simulink model "Arti_DeltaSM_Control_Fricc"  (R2014a)
settings: Solver=ode15s  StartTime=0.0  StopTime=6  FixedStep=0.0005  RelTol=1e-3
PreLoadFcn:
  | Fs=0.001;
  | Fc=0.0005;
undefined symbols (not defined in the file or in its folder): X, Y, Z
libraries: sm_lib x238, Fricciones x15, nesl_utility x10, simulink x3
(part 1 of 6)
Description:
  | Modelo de un robot tipo Delta, con:
  | -Fricción en las articulaciones
  | -Con interpolador de orden 5 en el espacio operacional.
  | -Cinematica inversa
  | -Sigue una trayectoria dada de pick and place con un control, y se obtiene la posicion final del efector.
  | -Tiene un control PID
  | 
  | le falta caracterizacion de los motores
settings Model: Creator=Sebastian Serna Palleja  LastModifiedBy=Sebastian
settings Model: ModifiedComment=|
  | Sebastian -- Mon Apr 11 18:51:16 2016 -- Version 1.58
  | actualizacion de pesos
settings Model: ModifiedHistory=|
  | Sebastian -- Mon Apr 11 18:51:16 2016 -- Version 1.58
  | actualizacion de pesos
  | 
  | Sebastian -- Sat Apr 09 23:12:04 2016 -- Version 1.56
  | Modelo organizado
settings SolverCC: MaxConsecutiveMinStep=4

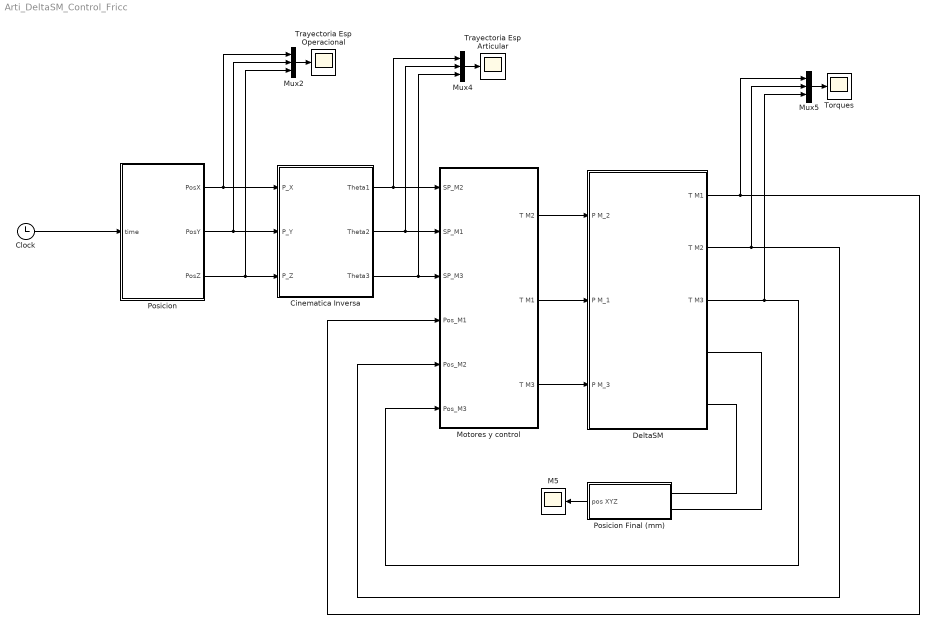
== system Arti_DeltaSM_Control_Fricc ==
  Cinematica Inversa : Subsystem
  Clock : Clock
  DeltaSM : Subsystem
  M5 : Scope
      settings: TimeRange=2  YMin=-450  YMax=50  SaveName=salida1
  Motores y control : Subsystem
  Mux2 : Mux  Inputs=3
  Mux4 : Mux  Inputs=3
  Mux5 : Mux  Inputs=3
  "Posicion " : MATLAB Function  TreatAsAtomicUnit=on
  Posicion Final (mm) : Subsystem
  Torques : Scope
      settings: SaveName=ScopeData11
  Trayectoria Esp Articular : Scope
      settings: SaveName=ScopeData9
  Trayectoria Esp Operacional : Scope
      settings: SaveName=ScopeData4
  wires:
  Posicion Final (mm)/1(pos XYZ) -> M5/1
  Clock/1 -> "Posicion "/1(time)
  Motores y control/3(T M3) -> DeltaSM/3(P M_3)
  Motores y control/2(T M1) -> DeltaSM/2(P M_1)
  Motores y control/1(T M2) -> DeltaSM/1(P M_2)
  Mux2/1 -> Trayectoria Esp Operacional/1
  "Posicion "/3(PosZ) -> Mux2/3, Cinematica Inversa/3(P_Z)
  "Posicion "/2(PosY) -> Mux2/2, Cinematica Inversa/2(P_Y)
  "Posicion "/1(PosX) -> Mux2/1, Cinematica Inversa/1(P_X)
  Mux4/1 -> Trayectoria Esp Articular/1
  Cinematica Inversa/3(Theta3) -> Mux4/3, Motores y control/3(SP_M3)
  Cinematica Inversa/2(Theta2) -> Mux4/2, Motores y control/2(SP_M1)
  Cinematica Inversa/1(Theta1) -> Mux4/1, Motores y control/1(SP_M2)
  Mux5/1 -> Torques/1
  DeltaSM/3(T M3) -> Mux5/3, Motores y control/6(Pos_M3)
  DeltaSM/2(T M2) -> Mux5/2, Motores y control/5(Pos_M2)
  DeltaSM/1(T M1) -> Mux5/1, Motores y control/4(Pos_M1)
  connections:
  Posicion Final (mm)/LConn2 -- DeltaSM/RConn1
  Posicion Final (mm)/LConn1 -- DeltaSM/RConn2

== system Arti_DeltaSM_Control_Fricc/Cinematica Inversa ==
  P_X : Inport
  P_Y : Inport  Port=2
  P_Z : Inport  Port=3
  Cinematica Inversa : MATLAB Function  TreatAsAtomicUnit=on
  G_1 : Gain
  G_2 : Gain
  G_3 : Gain  Gain=-1
  Retardo1 : TransportDelay  DelayTime=0.01
  Retardo2 : TransportDelay  DelayTime=0.01
  Retardo3 : TransportDelay  DelayTime=0.01
  Theta1 : Outport
  Theta2 : Outport  Port=2
  Theta3 : Outport  Port=3
  wires:
  P_X/1 -> Cinematica Inversa/1(Px)
  P_Y/1 -> Cinematica Inversa/2(Py)
  Cinematica Inversa/3(ThetaM3) -> G_3/1, Retardo1/1
  Retardo2/1 -> Cinematica Inversa/5(AntThetaM2)
  Retardo3/1 -> Cinematica Inversa/4(AntThetaM1)
  Retardo1/1 -> Cinematica Inversa/6(AntThetaM3)
  Cinematica Inversa/1(ThetaM1) -> G_1/1, Retardo3/1
  Cinematica Inversa/2(ThetaM2) -> G_2/1, Retardo2/1
  G_1/1 -> Theta1/1
  G_2/1 -> Theta2/1
  G_3/1 -> Theta3/1
  P_Z/1 -> Cinematica Inversa/3(Pz)

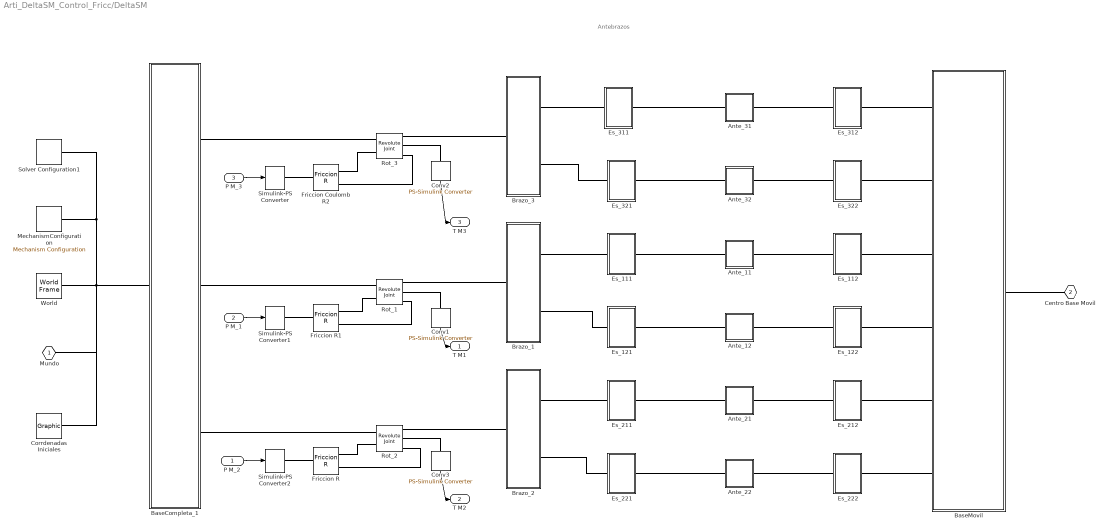
== system Arti_DeltaSM_Control_Fricc/DeltaSM ==
  note: Antebrazos
  P M_2 : Inport
  P M_1 : Inport  Port=2
  P M_3 : Inport  Port=3
  Ante_11 : Subsystem
  Ante_12 : Subsystem
  Ante_21 : Subsystem
  Ante_22 : Subsystem
  Ante_31 : Subsystem
  Ante_32 : Subsystem
  BaseCompleta_1 : Subsystem
  BaseMovil : Subsystem
  Brazo_1 : Subsystem
  Brazo_2 : Subsystem
  Brazo_3 : Subsystem
  Conv1 : nesl_utility/PS-Simulink Converter  PhysicalDomain=network_engine_domain  SubClassName=ps_output  LeftPortType=input  RightPortType=output  PseudoPeriodic=off  Frequencies=[]  Unit=rad  AffineConversion=off
  Conv2 : nesl_utility/PS-Simulink Converter  PhysicalDomain=network_engine_domain  SubClassName=ps_output  LeftPortType=input  RightPortType=output  PseudoPeriodic=off  Frequencies=[]  Unit=rad  AffineConversion=off
  Conv3 : nesl_utility/PS-Simulink Converter  PhysicalDomain=network_engine_domain  SubClassName=ps_output  LeftPortType=input  RightPortType=output  PseudoPeriodic=off  Frequencies=[]  Unit=rad  AffineConversion=off
  "Corrdenadas Iniciales " : sm_lib/Body Elements/Graphic  GraphicType=Marker  MarkerShape=Frame  MarkerSize=25  MarkerSizeUnits=m  GraphicVisPropType=SimpleVisualProperties  GraphicDiffuseColor=[0.0 0.0 0.0]  GraphicSpecularColor=[0.2 0.2 0.2]  GraphicAmbientColor=[0.5 0.5 0.5]  GraphicEmissiveColor=[0.0 0.0 0.0 1.0]  GraphicShininess=24.0  GraphicOpacity=1.0  BlockFunction=simmechanics.library.body_elements.graphic
  Es_111 : Subsystem
  Es_112 : Subsystem
  Es_121 : Subsystem
  Es_122 : Subsystem
  Es_211 : Subsystem
  Es_212 : Subsystem
  Es_221 : Subsystem
  Es_222 : Subsystem
  Es_311 : Subsystem
  Es_312 : Subsystem
  Es_321 : Subsystem
  Es_322 : Subsystem
  Friccion Coulomb R2 : Fricciones/Friccion R
  Friccion R : Fricciones/Friccion R
  Friccion R1 : Fricciones/Friccion R
  MechanismConfiguration : sm_lib/Utilities/Mechanism Configuration  UniformGravity=Constant  GravityVector=[0 0 -9.81]  GravityUnits=m/s^2  LinearizationDelta=0.001  BlockFunction=simmechanics.library.utilities.mechanism_configuration
  Rot_1 : sm_lib/Joints/Revolute Joint  SenseConstraintForce=off  SenseConstraintForceX=off  SenseConstraintForceY=off  SenseConstraintForceZ=off  SenseConstraintTorque=off  SenseConstraintTorqueX=off  SenseConstraintTorqueY=off  SenseConstraintTorqueZ=off  SenseTotalForce=off  SenseTotalForceX=off  SenseTotalForceY=off  SenseTotalForceZ=off  SenseTotalTorque=off  SenseTotalTorqueX=off  SenseTotalTorqueY=off  SenseTotalTorqueZ=off  CompositeWrenchDir=FollowerOnBase  CompositeWrenchFrame=BaseFrame  EquilibriumPosition=0  EquilibriumPositionUnits=rad  SpringStiffness=0  SpringStiffnessUnits=m*N/rad  DampingCoefficient=0  DampingCoefficientUnits=m*s*N/rad  TorqueActuationMode=InputTorque  MotionActuationMode=ComputedMotion  SensePosition=on  SenseVelocity=on  SenseAcceleration=off  SenseTorqueForce=off  PositionTargetValue=90  PositionTargetValueUnits=deg  PositionTargetSpecify=on  PositionTargetPriority=High  VelocityTargetValue=0  VelocityTargetValueUnits=deg/s  VelocityTargetSpecify=off  VelocityTargetPriority=High  BlockFunction=simmechanics.library.joints.revolute_joint
  Rot_2 : sm_lib/Joints/Revolute Joint  SenseConstraintForce=off  SenseConstraintForceX=off  SenseConstraintForceY=off  SenseConstraintForceZ=off  SenseConstraintTorque=off  SenseConstraintTorqueX=off  SenseConstraintTorqueY=off  SenseConstraintTorqueZ=off  SenseTotalForce=off  SenseTotalForceX=off  SenseTotalForceY=off  SenseTotalForceZ=off  SenseTotalTorque=off  SenseTotalTorqueX=off  SenseTotalTorqueY=off  SenseTotalTorqueZ=off  CompositeWrenchDir=FollowerOnBase  CompositeWrenchFrame=BaseFrame  EquilibriumPosition=0  EquilibriumPositionUnits=rad  SpringStiffness=0  SpringStiffnessUnits=m*N/rad  DampingCoefficient=0  DampingCoefficientUnits=m*s*N/rad  TorqueActuationMode=InputTorque  MotionActuationMode=ComputedMotion  SensePosition=on  SenseVelocity=on  SenseAcceleration=off  SenseTorqueForce=off  PositionTargetValue=90  PositionTargetValueUnits=deg  PositionTargetSpecify=on  PositionTargetPriority=High  VelocityTargetValue=0  VelocityTargetValueUnits=deg/s  VelocityTargetSpecify=off  VelocityTargetPriority=High  BlockFunction=simmechanics.library.joints.revolute_joint
  Rot_3 : sm_lib/Joints/Revolute Joint  SenseConstraintForce=off  SenseConstraintForceX=off  SenseConstraintForceY=off  SenseConstraintForceZ=off  SenseConstraintTorque=off  SenseConstraintTorqueX=off  SenseConstraintTorqueY=off  SenseConstraintTorqueZ=off  SenseTotalForce=off  SenseTotalForceX=off  SenseTotalForceY=off  SenseTotalForceZ=off  SenseTotalTorque=off  SenseTotalTorqueX=off  SenseTotalTorqueY=off  SenseTotalTorqueZ=off  CompositeWrenchDir=FollowerOnBase  CompositeWrenchFrame=BaseFrame  EquilibriumPosition=0  EquilibriumPositionUnits=rad  SpringStiffness=0  SpringStiffnessUnits=m*N/rad  DampingCoefficient=0  DampingCoefficientUnits=m*s*N/rad  TorqueActuationMode=InputTorque  MotionActuationMode=ComputedMotion  SensePosition=on  SenseVelocity=on  SenseAcceleration=off  SenseTorqueForce=off  PositionTargetValue=-90  PositionTargetValueUnits=deg  PositionTargetSpecify=on  PositionTargetPriority=High  VelocityTargetValue=0  VelocityTargetValueUnits=deg/s  VelocityTargetSpecify=off  VelocityTargetPriority=High  BlockFunction=simmechanics.library.joints.revolute_joint
  Simulink-PS Converter : nesl_utility/Simulink-PS Converter  PhysicalDomain=network_engine_domain  SubClassName=ps_input  LeftPortType=input  RightPortType=output  PseudoPeriodic=off  Frequencies=[]  NoiseDistribution=none  NoiseParameters=[]  Unit=N*m  AffineConversion=off  InputFiltering=off  SimscapeFilterOrder=1  InputFilterTimeConstant=0.001  UdotUserProvided=1
  Simulink-PS Converter1 : nesl_utility/Simulink-PS Converter  PhysicalDomain=network_engine_domain  SubClassName=ps_input  LeftPortType=input  RightPortType=output  PseudoPeriodic=off  Frequencies=[]  NoiseDistribution=none  NoiseParameters=[]  Unit=N*m  AffineConversion=off  InputFiltering=off  SimscapeFilterOrder=1  InputFilterTimeConstant=0.001  UdotUserProvided=1
  Simulink-PS Converter2 : nesl_utility/Simulink-PS Converter  PhysicalDomain=network_engine_domain  SubClassName=ps_input  LeftPortType=input  RightPortType=output  PseudoPeriodic=off  Frequencies=[]  NoiseDistribution=none  NoiseParameters=[]  Unit=N*m  AffineConversion=off  InputFiltering=off  SimscapeFilterOrder=1  InputFilterTimeConstant=0.001  UdotUserProvided=1
  Solver Configuration1 : nesl_utility/Solver Configuration  PhysicalDomain=network_engine_domain  SubClassName=solver  LeftPortType=input  RightPortType=generic  Accelerate=off  Tones=[]  Harmonics=[]  SimulateNoise=off  Profile=off  UseLocalSampling=off  EnableSwitchedLinearOptims=on  FrequencyDomain=off  UseCCode=off  RelTol=0.001  AbsTol=1e-06  MinStep=1e-09  ToWorkspace=off  DoDC=on  ResidualTolerance=1e-09  UseLocalSolver=off  LocalSolverChoice=NE_BACKWARD_EULER_ADVANCER  LocalSolverSampleTime=0.00001  DoFixedCost=off  MaxNonlinIter=30  MaxModeIter=2  LinearAlgebra=Full  DelaysMemoryBudget=2048  AutomaticFiltering=on  FilteringTimeConstant=0.001
  World : sm_lib/Frames and Transforms/World Frame  BlockFunction=simmechanics.library.frames_transforms.world_frame
  Mundo : PMIOPort  Port=1  Side=Right
  Centro Base Movil : PMIOPort  Priority=1  Port=2  Side=Right
  T M1 : Outport
  T M2 : Outport  Port=2
  T M3 : Outport  Port=3
  wires:
  Conv2/1 -> T M3/1
  Conv1/1 -> T M1/1
  Conv3/1 -> T M2/1
  P M_1/1 -> Simulink-PS Converter1/1
  P M_3/1 -> Simulink-PS Converter/1
  P M_2/1 -> Simulink-PS Converter2/1
  connections:
  BaseCompleta_1/RConn2 -- Rot_1/LConn1
  Brazo_2/LConn1 -- Rot_2/RConn1
  BaseCompleta_1/RConn1 -- Rot_3/LConn1
  Brazo_3/LConn1 -- Rot_3/RConn1
  Brazo_1/LConn1 -- Rot_1/RConn1
  BaseCompleta_1/RConn3 -- Rot_2/LConn1
  Conv2/LConn1 -- Rot_3/RConn2
  Conv1/LConn1 -- Rot_1/RConn2
  Conv3/LConn1 -- Rot_2/RConn2
  BaseMovil/RConn1 -- Centro Base Movil/RConn1
  Friccion R1/LConn1 -- Simulink-PS Converter1/RConn1
  Friccion R1/RConn1 -- Rot_1/LConn2
  Friccion R1/RConn2 -- Rot_1/RConn3
  Friccion R/RConn2 -- Rot_2/RConn3
  Rot_3/RConn3 -- Friccion Coulomb R2/RConn2
  Friccion R/LConn1 -- Simulink-PS Converter2/RConn1
  Friccion R/RConn1 -- Rot_2/LConn2
  Friccion Coulomb R2/RConn1 -- Rot_3/LConn2
  Simulink-PS Converter/RConn1 -- Friccion Coulomb R2/LConn1
  Ante_11/RConn1 -- Es_112/LConn1
  Ante_22/LConn1 -- Es_221/RConn1
  Ante_31/RConn1 -- Es_312/LConn1
  Brazo_1/RConn2 -- Es_121/LConn1
  Brazo_3/RConn2 -- Es_321/LConn1
  Ante_32/RConn1 -- Es_322/LConn1
  Ante_22/RConn1 -- Es_222/LConn1
  Brazo_3/RConn1 -- Es_311/LConn1
  Ante_21/LConn1 -- Es_211/RConn1
  Ante_12/RConn1 -- Es_122/LConn1
  Ante_31/LConn1 -- Es_311/RConn1
  Ante_11/LConn1 -- Es_111/RConn1
  Ante_21/RConn1 -- Es_212/LConn1
  BaseMovil/LConn1 -- Es_312/RConn1
  BaseMovil/LConn5 -- Es_212/RConn1
  BaseMovil/LConn6 -- Es_222/RConn1
  Ante_32/LConn1 -- Es_321/RConn1
  BaseMovil/LConn3 -- Es_112/RConn1
  Brazo_2/RConn2 -- Es_221/LConn1
  BaseMovil/LConn4 -- Es_122/RConn1
  BaseMovil/LConn2 -- Es_322/RConn1
  Brazo_2/RConn1 -- Es_211/LConn1
  Ante_12/LConn1 -- Es_121/RConn1
  Brazo_1/RConn1 -- Es_111/LConn1
  Solver Configuration1/RConn1 -- MechanismConfiguration/RConn1 -- BaseCompleta_1/LConn1 -- Mundo/RConn1 -- "Corrdenadas Iniciales "/RConn1 -- World/RConn1

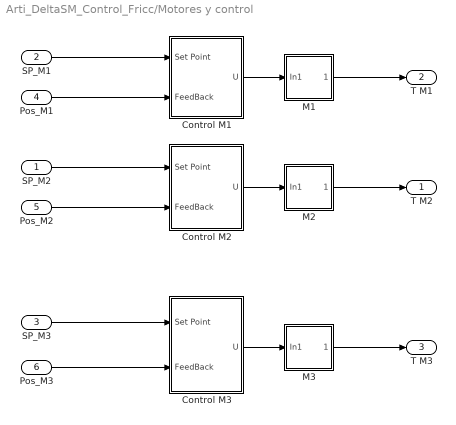
== system Arti_DeltaSM_Control_Fricc/Motores y control ==
  SP_M2 : Inport
  SP_M1 : Inport  Port=2
  SP_M3 : Inport  Port=3
  Pos_M1 : Inport  Port=4
  Pos_M2 : Inport  Port=5
  Pos_M3 : Inport  Port=6
  Control M1 : Subsystem
  Control M2 : Subsystem
  Control M3 : Subsystem
  M1 : Subsystem
  M2 : Subsystem
  M3 : Subsystem
  T M2 : Outport
  T M1 : Outport  Port=2
  T M3 : Outport  Port=3
  wires:
  SP_M2/1 -> Control M2/1(Set Point)
  Pos_M2/1 -> Control M2/2(FeedBack)
  SP_M1/1 -> Control M1/1(Set Point)
  Pos_M1/1 -> Control M1/2(FeedBack)
  Control M2/1(U) -> M2/1(In1)
  Control M1/1(U) -> M1/1(In1)
  Control M3/1(U) -> M3/1(In1)
  SP_M3/1 -> Control M3/1(Set Point)
  Pos_M3/1 -> Control M3/2(FeedBack)
  M1/1(Out1) -> T M1/1
  M2/1(Out1) -> T M2/1
  M3/1(Out1) -> T M3/1

== system Arti_DeltaSM_Control_Fricc/Posicion Final (mm) ==
  M1 : Scope
      settings: SaveName=ScopeData7
  M2 : Scope
      settings: SaveName=ScopeData8
  "M3 " : Scope
      settings: SaveName=ScopeData6
  Mux : Mux  Inputs=3
  Pos X Converter : nesl_utility/PS-Simulink Converter  PhysicalDomain=network_engine_domain  SubClassName=ps_output  LeftPortType=input  RightPortType=output  PseudoPeriodic=off  Frequencies=[]  Unit=mm  AffineConversion=off
  Pos Y Converter1 : nesl_utility/PS-Simulink Converter  PhysicalDomain=network_engine_domain  SubClassName=ps_output  LeftPortType=input  RightPortType=output  PseudoPeriodic=off  Frequencies=[]  Unit=mm  AffineConversion=off
  Pos Z Converter2 : nesl_utility/PS-Simulink Converter  PhysicalDomain=network_engine_domain  SubClassName=ps_output  LeftPortType=input  RightPortType=output  PseudoPeriodic=off  Frequencies=[]  Unit=mm  AffineConversion=off
  Transform Sensor : sm_lib/Frames and Transforms/Transform Sensor  MeasurementFrame=World  SenseAngle=off  SenseAxis=off  SenseAngle1=off  SenseAngle2=off  SenseAngle3=off  SenseQ=off  SenseR=off  SenseOmegaX=off  SenseOmegaY=off  SenseOmegaZ=off  SenseOmega1=off  SenseOmega2=off  SenseOmega3=off  SenseQDot=off  SenseRDot=off  SenseAlphaX=off  SenseAlphaY=off  SenseAlphaZ=off  SenseAlpha1=off  SenseAlpha2=off  SenseAlpha3=off  SenseQDDot=off  SenseRDDot=off  SenseX=on  SenseY=on  SenseZ=on  SenseRad=off  SenseAzim=off  SenseDist=off  SenseInc=off  SenseXDot=off  SenseYDot=off  SenseZDot=off  SenseRadDot=off  SenseAzimDot=off  SenseDistDot=off  SenseIncDot=off  SenseXDDot=off  SenseYDDot=off  SenseZDDot=off  SenseRadDDot=off  SenseAzimDDot=off  SenseDistDDot=off  SenseIncDDot=off  BlockFunction=simmechanics.library.frames_transforms.transform_sensor
  Centro Base Movil : PMIOPort  Port=1  Side=Left
  world : PMIOPort  Port=2  Side=Left
  pos XYZ : Outport
  wires:
  Pos Z Converter2/1 -> M2/1, Mux/3
  Mux/1 -> pos XYZ/1
  Pos Y Converter1/1 -> Mux/2, M1/1
  Pos X Converter/1 -> "M3 "/1, Mux/1
  connections:
  world/RConn1 -- Transform Sensor/LConn1
  Pos Z Converter2/LConn1 -- Transform Sensor/RConn4
  Transform Sensor/RConn2 -- Pos X Converter/LConn1
  Pos Y Converter1/LConn1 -- Transform Sensor/RConn3
  Centro Base Movil/RConn1 -- Transform Sensor/RConn1

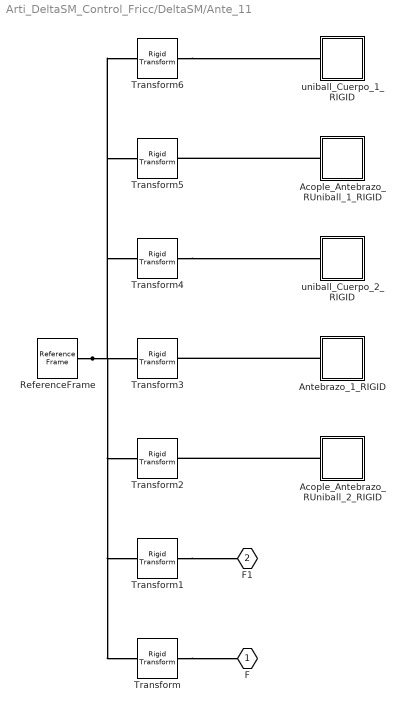
== system Arti_DeltaSM_Control_Fricc/DeltaSM/Ante_11 ==
  Acople_Antebrazo_RUniball_1_RIGID : Subsystem
  Acople_Antebrazo_RUniball_2_RIGID : Subsystem
  Antebrazo_1_RIGID : Subsystem
  ReferenceFrame : sm_lib/Frames and Transforms/Reference Frame  BlockFunction=simmechanics.library.frames_transforms.reference_frame
  Transform : sm_lib/Frames and Transforms/Rigid Transform  TranslationMethod=Cartesian  TranslationLengthUnit=mm  TranslationStandardAxis=+Z  TranslationStandardOffset=0  TranslationCartesianOffset=[-16.089268306127384 11.758961591624281 40.649351392904187]  TranslationROffset=0  TranslationROffsetUnits=m  TranslationZOffset=0  TranslationZOffsetUnits=m  TranslationThetaOffset=0  TranslationThetaOffsetUnits=deg  RotationMethod=ArbitraryAxis  RotationAngleUnits=rad  RotationStandardAxis=+Z  RotationAngle=0  RotationArbitraryAxis=[0 0 0]  FollAlignAxisA=+X  BaseAlignAxisA=+Y  FollAlignAxisB=+Y  BaseAlignAxisB=+Z  BlockFunction=simmechanics.library.frames_transforms.rigid_transform
  Transform1 : sm_lib/Frames and Transforms/Rigid Transform  TranslationMethod=Cartesian  TranslationLengthUnit=mm  TranslationStandardAxis=+Z  TranslationStandardOffset=0  TranslationCartesianOffset=[-16.089268306127369 -263.24103840837563 40.649351392904151]  TranslationROffset=0  TranslationROffsetUnits=m  TranslationZOffset=0  TranslationZOffsetUnits=m  TranslationThetaOffset=0  TranslationThetaOffsetUnits=deg  RotationMethod=ArbitraryAxis  RotationAngleUnits=rad  RotationStandardAxis=+Z  RotationAngle=0  RotationArbitraryAxis=[0 0 0]  FollAlignAxisA=+X  BaseAlignAxisA=+Y  FollAlignAxisB=+Y  BaseAlignAxisB=+Z  BlockFunction=simmechanics.library.frames_transforms.rigid_transform
  Transform2 : sm_lib/Frames and Transforms/Rigid Transform  TranslationMethod=Cartesian  TranslationLengthUnit=mm  TranslationStandardAxis=+Z  TranslationStandardOffset=0  TranslationCartesianOffset=[-16.089268306127376 -51.741038408375687 40.649351392904165]  TranslationROffset=0  TranslationROffsetUnits=m  TranslationZOffset=0  TranslationZOffsetUnits=m  TranslationThetaOffset=0  TranslationThetaOffsetUnits=deg  RotationMethod=ArbitraryAxis  RotationAngleUnits=rad  RotationStandardAxis=+Z  RotationAngle=2.7352803968007873  RotationArbitraryAxis=[-0.2059979679735047 0.69194105138761164 0.69194105138761175]  FollAlignAxisA=+X  BaseAlignAxisA=+Y  FollAlignAxisB=+Y  BaseAlignAxisB=+Z  BlockFunction=simmechanics.library.frames_transforms.rigid_transform
  Transform3 : sm_lib/Frames and Transforms/Rigid Transform  TranslationMethod=Cartesian  TranslationLengthUnit=mm  TranslationStandardAxis=+Z  TranslationStandardOffset=0  TranslationCartesianOffset=[-16.089268306127384 -227.74103840837574 40.64935139290418]  TranslationROffset=0  TranslationROffsetUnits=m  TranslationZOffset=0  TranslationZOffsetUnits=m  TranslationThetaOffset=0  TranslationThetaOffsetUnits=deg  RotationMethod=ArbitraryAxis  RotationAngleUnits=rad  RotationStandardAxis=+Z  RotationAngle=2.7352803968007873  RotationArbitraryAxis=[-0.2059979679735047 0.69194105138761164 0.69194105138761175]  FollAlignAxisA=+X  BaseAlignAxisA=+Y  FollAlignAxisB=+Y  BaseAlignAxisB=+Z  BlockFunction=simmechanics.library.frames_transforms.rigid_transform
  Transform4 : sm_lib/Frames and Transforms/Rigid Transform  TranslationMethod=Cartesian  TranslationLengthUnit=mm  TranslationStandardAxis=+Z  TranslationStandardOffset=0  TranslationCartesianOffset=[-16.089268306127369 -263.24103840837563 40.649351392904151]  TranslationROffset=0  TranslationROffsetUnits=m  TranslationZOffset=0  TranslationZOffsetUnits=m  TranslationThetaOffset=0  TranslationThetaOffsetUnits=deg  RotationMethod=ArbitraryAxis  RotationAngleUnits=rad  RotationStandardAxis=+Z  RotationAngle=3.1415926535897931  RotationArbitraryAxis=[-1.1188966420050406e-16 0 1]  FollAlignAxisA=+X  BaseAlignAxisA=+Y  FollAlignAxisB=+Y  BaseAlignAxisB=+Z  BlockFunction=simmechanics.library.frames_transforms.rigid_transform
  Transform5 : sm_lib/Frames and Transforms/Rigid Transform  TranslationMethod=Cartesian  TranslationLengthUnit=mm  TranslationStandardAxis=+Z  TranslationStandardOffset=0  TranslationCartesianOffset=[-16.089268306127391 -199.7410384083758 40.64935139290418]  TranslationROffset=0  TranslationROffsetUnits=m  TranslationZOffset=0  TranslationZOffsetUnits=m  TranslationThetaOffset=0  TranslationThetaOffsetUnits=deg  RotationMethod=ArbitraryAxis  RotationAngleUnits=rad  RotationStandardAxis=+Z  RotationAngle=2.7352803968007873  RotationArbitraryAxis=[0.2059979679735047 0.69194105138761164 -0.69194105138761175]  FollAlignAxisA=+X  BaseAlignAxisA=+Y  FollAlignAxisB=+Y  BaseAlignAxisB=+Z  BlockFunction=simmechanics.library.frames_transforms.rigid_transform
  Transform6 : sm_lib/Frames and Transforms/Rigid Transform  TranslationMethod=Cartesian  TranslationLengthUnit=mm  TranslationStandardAxis=+Z  TranslationStandardOffset=0  TranslationCartesianOffset=[-16.089268306127376 11.758961591624317 40.649351392904165]  TranslationROffset=0  TranslationROffsetUnits=m  TranslationZOffset=0  TranslationZOffsetUnits=m  TranslationThetaOffset=0  TranslationThetaOffsetUnits=deg  RotationMethod=None  RotationAngleUnits=deg  RotationStandardAxis=+Z  RotationAngle=0  RotationArbitraryAxis=[0 0 1]  FollAlignAxisA=+X  BaseAlignAxisA=+Y  FollAlignAxisB=+Y  BaseAlignAxisB=+Z  BlockFunction=simmechanics.library.frames_transforms.rigid_transform
  uniball_Cuerpo_1_RIGID : Subsystem
  uniball_Cuerpo_2_RIGID : Subsystem
  F : PMIOPort  Port=1  Side=Left
  F1 : PMIOPort  Port=2  Side=Right
  connections:
  ReferenceFrame/RConn1 -- Transform/LConn1 -- Transform1/LConn1 -- Transform2/LConn1 -- Transform3/LConn1 -- Transform4/LConn1 -- Transform5/LConn1 -- Transform6/LConn1
  Transform/RConn1 -- F/RConn1
  Transform1/RConn1 -- F1/RConn1
  Acople_Antebrazo_RUniball_2_RIGID/LConn1 -- Transform2/RConn1
  Antebrazo_1_RIGID/LConn1 -- Transform3/RConn1
  Transform4/RConn1 -- uniball_Cuerpo_2_RIGID/LConn1
  Acople_Antebrazo_RUniball_1_RIGID/LConn1 -- Transform5/RConn1
  Transform6/RConn1 -- uniball_Cuerpo_1_RIGID/LConn1

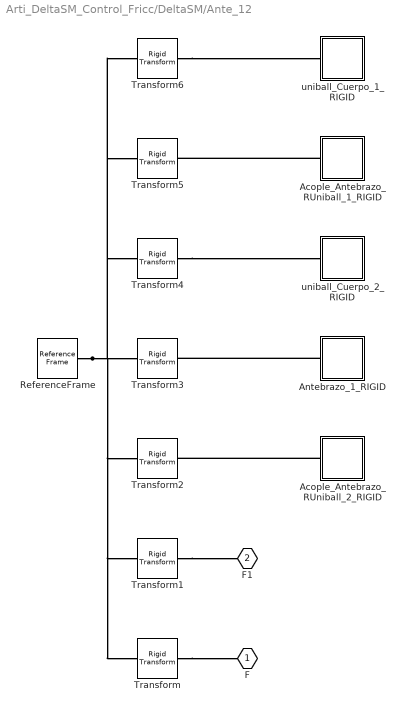
== system Arti_DeltaSM_Control_Fricc/DeltaSM/Ante_12 ==
  Acople_Antebrazo_RUniball_1_RIGID : Subsystem
  Acople_Antebrazo_RUniball_2_RIGID : Subsystem
  Antebrazo_1_RIGID : Subsystem
  ReferenceFrame : sm_lib/Frames and Transforms/Reference Frame  BlockFunction=simmechanics.library.frames_transforms.reference_frame
  Transform : sm_lib/Frames and Transforms/Rigid Transform  TranslationMethod=Cartesian  TranslationLengthUnit=mm  TranslationStandardAxis=+Z  TranslationStandardOffset=0  TranslationCartesianOffset=[-16.089268306127394 11.758961591624296 40.64935139290418]  TranslationROffset=0  TranslationROffsetUnits=m  TranslationZOffset=0  TranslationZOffsetUnits=m  TranslationThetaOffset=0  TranslationThetaOffsetUnits=deg  RotationMethod=ArbitraryAxis  RotationAngleUnits=rad  RotationStandardAxis=+Z  RotationAngle=0  RotationArbitraryAxis=[0 0 0]  FollAlignAxisA=+X  BaseAlignAxisA=+Y  FollAlignAxisB=+Y  BaseAlignAxisB=+Z  BlockFunction=simmechanics.library.frames_transforms.rigid_transform
  Transform1 : sm_lib/Frames and Transforms/Rigid Transform  TranslationMethod=Cartesian  TranslationLengthUnit=mm  TranslationStandardAxis=+Z  TranslationStandardOffset=0  TranslationCartesianOffset=[-16.089268306127391 -263.24103840837574 40.649351392904165]  TranslationROffset=0  TranslationROffsetUnits=m  TranslationZOffset=0  TranslationZOffsetUnits=m  TranslationThetaOffset=0  TranslationThetaOffsetUnits=deg  RotationMethod=ArbitraryAxis  RotationAngleUnits=rad  RotationStandardAxis=+Z  RotationAngle=0  RotationArbitraryAxis=[0 0 0]  FollAlignAxisA=+X  BaseAlignAxisA=+Y  FollAlignAxisB=+Y  BaseAlignAxisB=+Z  BlockFunction=simmechanics.library.frames_transforms.rigid_transform
  Transform2 : sm_lib/Frames and Transforms/Rigid Transform  TranslationMethod=Cartesian  TranslationLengthUnit=mm  TranslationStandardAxis=+Z  TranslationStandardOffset=0  TranslationCartesianOffset=[-16.089268306127362 -51.741038408375672 40.64935139290418]  TranslationROffset=0  TranslationROffsetUnits=m  TranslationZOffset=0  TranslationZOffsetUnits=m  TranslationThetaOffset=0  TranslationThetaOffsetUnits=deg  RotationMethod=ArbitraryAxis  RotationAngleUnits=rad  RotationStandardAxis=+Z  RotationAngle=2.7352803968007873  RotationArbitraryAxis=[-0.20599796797350473 0.69194105138761164 0.69194105138761175]  FollAlignAxisA=+X  BaseAlignAxisA=+Y  FollAlignAxisB=+Y  BaseAlignAxisB=+Z  BlockFunction=simmechanics.library.frames_transforms.rigid_transform
  Transform3 : sm_lib/Frames and Transforms/Rigid Transform  TranslationMethod=Cartesian  TranslationLengthUnit=mm  TranslationStandardAxis=+Z  TranslationStandardOffset=0  TranslationCartesianOffset=[-16.089268306127376 -227.74103840837577 40.64935139290418]  TranslationROffset=0  TranslationROffsetUnits=m  TranslationZOffset=0  TranslationZOffsetUnits=m  TranslationThetaOffset=0  TranslationThetaOffsetUnits=deg  RotationMethod=ArbitraryAxis  RotationAngleUnits=rad  RotationStandardAxis=+Z  RotationAngle=2.7352803968007873  RotationArbitraryAxis=[-0.20599796797350473 0.69194105138761164 0.69194105138761175]  FollAlignAxisA=+X  BaseAlignAxisA=+Y  FollAlignAxisB=+Y  BaseAlignAxisB=+Z  BlockFunction=simmechanics.library.frames_transforms.rigid_transform
  Transform4 : sm_lib/Frames and Transforms/Rigid Transform  TranslationMethod=Cartesian  TranslationLengthUnit=mm  TranslationStandardAxis=+Z  TranslationStandardOffset=0  TranslationCartesianOffset=[-16.089268306127391 -263.24103840837574 40.649351392904165]  TranslationROffset=0  TranslationROffsetUnits=m  TranslationZOffset=0  TranslationZOffsetUnits=m  TranslationThetaOffset=0  TranslationThetaOffsetUnits=deg  RotationMethod=ArbitraryAxis  RotationAngleUnits=rad  RotationStandardAxis=+Z  RotationAngle=3.1415926535897931  RotationArbitraryAxis=[-1.1188966420050406e-16 0 1]  FollAlignAxisA=+X  BaseAlignAxisA=+Y  FollAlignAxisB=+Y  BaseAlignAxisB=+Z  BlockFunction=simmechanics.library.frames_transforms.rigid_transform
  Transform5 : sm_lib/Frames and Transforms/Rigid Transform  TranslationMethod=Cartesian  TranslationLengthUnit=mm  TranslationStandardAxis=+Z  TranslationStandardOffset=0  TranslationCartesianOffset=[-16.089268306127376 -199.74103840837577 40.649351392904165]  TranslationROffset=0  TranslationROffsetUnits=m  TranslationZOffset=0  TranslationZOffsetUnits=m  TranslationThetaOffset=0  TranslationThetaOffsetUnits=deg  RotationMethod=ArbitraryAxis  RotationAngleUnits=rad  RotationStandardAxis=+Z  RotationAngle=2.7352803968007873  RotationArbitraryAxis=[0.20599796797350473 0.69194105138761164 -0.69194105138761175]  FollAlignAxisA=+X  BaseAlignAxisA=+Y  FollAlignAxisB=+Y  BaseAlignAxisB=+Z  BlockFunction=simmechanics.library.frames_transforms.rigid_transform
  Transform6 : sm_lib/Frames and Transforms/Rigid Transform  TranslationMethod=Cartesian  TranslationLengthUnit=mm  TranslationStandardAxis=+Z  TranslationStandardOffset=0  TranslationCartesianOffset=[-16.089268306127376 11.758961591624317 40.649351392904165]  TranslationROffset=0  TranslationROffsetUnits=m  TranslationZOffset=0  TranslationZOffsetUnits=m  TranslationThetaOffset=0  TranslationThetaOffsetUnits=deg  RotationMethod=None  RotationAngleUnits=deg  RotationStandardAxis=+Z  RotationAngle=0  RotationArbitraryAxis=[0 0 1]  FollAlignAxisA=+X  BaseAlignAxisA=+Y  FollAlignAxisB=+Y  BaseAlignAxisB=+Z  BlockFunction=simmechanics.library.frames_transforms.rigid_transform
  uniball_Cuerpo_1_RIGID : Subsystem
  uniball_Cuerpo_2_RIGID : Subsystem
  F : PMIOPort  Port=1  Side=Left
  F1 : PMIOPort  Port=2  Side=Right
  connections:
  ReferenceFrame/RConn1 -- Transform/LConn1 -- Transform1/LConn1 -- Transform2/LConn1 -- Transform3/LConn1 -- Transform4/LConn1 -- Transform5/LConn1 -- Transform6/LConn1
  Transform/RConn1 -- F/RConn1
  Transform1/RConn1 -- F1/RConn1
  Acople_Antebrazo_RUniball_2_RIGID/LConn1 -- Transform2/RConn1
  Antebrazo_1_RIGID/LConn1 -- Transform3/RConn1
  Transform4/RConn1 -- uniball_Cuerpo_2_RIGID/LConn1
  Acople_Antebrazo_RUniball_1_RIGID/LConn1 -- Transform5/RConn1
  Transform6/RConn1 -- uniball_Cuerpo_1_RIGID/LConn1

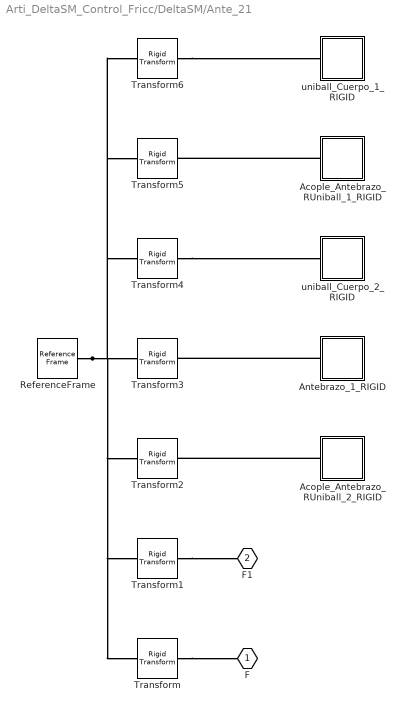
== system Arti_DeltaSM_Control_Fricc/DeltaSM/Ante_21 ==
  Acople_Antebrazo_RUniball_1_RIGID : Subsystem
  Acople_Antebrazo_RUniball_2_RIGID : Subsystem
  Antebrazo_1_RIGID : Subsystem
  ReferenceFrame : sm_lib/Frames and Transforms/Reference Frame  BlockFunction=simmechanics.library.frames_transforms.reference_frame
  Transform : sm_lib/Frames and Transforms/Rigid Transform  TranslationMethod=Cartesian  TranslationLengthUnit=mm  TranslationStandardAxis=+Z  TranslationStandardOffset=0  TranslationCartesianOffset=[-16.089268306127366 11.758961591624313 40.649351392904201]  TranslationROffset=0  TranslationROffsetUnits=m  TranslationZOffset=0  TranslationZOffsetUnits=m  TranslationThetaOffset=0  TranslationThetaOffsetUnits=deg  RotationMethod=ArbitraryAxis  RotationAngleUnits=rad  RotationStandardAxis=+Z  RotationAngle=0  RotationArbitraryAxis=[0 0 0]  FollAlignAxisA=+X  BaseAlignAxisA=+Y  FollAlignAxisB=+Y  BaseAlignAxisB=+Z  BlockFunction=simmechanics.library.frames_transforms.rigid_transform
  Transform1 : sm_lib/Frames and Transforms/Rigid Transform  TranslationMethod=Cartesian  TranslationLengthUnit=mm  TranslationStandardAxis=+Z  TranslationStandardOffset=0  TranslationCartesianOffset=[-16.089268306127362 -263.24103840837574 40.649351392904165]  TranslationROffset=0  TranslationROffsetUnits=m  TranslationZOffset=0  TranslationZOffsetUnits=m  TranslationThetaOffset=0  TranslationThetaOffsetUnits=deg  RotationMethod=ArbitraryAxis  RotationAngleUnits=rad  RotationStandardAxis=+Z  RotationAngle=0  RotationArbitraryAxis=[0 0 0]  FollAlignAxisA=+X  BaseAlignAxisA=+Y  FollAlignAxisB=+Y  BaseAlignAxisB=+Z  BlockFunction=simmechanics.library.frames_transforms.rigid_transform
  Transform2 : sm_lib/Frames and Transforms/Rigid Transform  TranslationMethod=Cartesian  TranslationLengthUnit=mm  TranslationStandardAxis=+Z  TranslationStandardOffset=0  TranslationCartesianOffset=[-16.089268306127376 -51.741038408375708 40.649351392904165]  TranslationROffset=0  TranslationROffsetUnits=m  TranslationZOffset=0  TranslationZOffsetUnits=m  TranslationThetaOffset=0  TranslationThetaOffsetUnits=deg  RotationMethod=ArbitraryAxis  RotationAngleUnits=rad  RotationStandardAxis=+Z  RotationAngle=2.7352803968007873  RotationArbitraryAxis=[-0.20599796797350473 0.69194105138761164 0.69194105138761175]  FollAlignAxisA=+X  BaseAlignAxisA=+Y  FollAlignAxisB=+Y  BaseAlignAxisB=+Z  BlockFunction=simmechanics.library.frames_transforms.rigid_transform
  Transform3 : sm_lib/Frames and Transforms/Rigid Transform  TranslationMethod=Cartesian  TranslationLengthUnit=mm  TranslationStandardAxis=+Z  TranslationStandardOffset=0  TranslationCartesianOffset=[-16.089268306127362 -227.74103840837572 40.649351392904173]  TranslationROffset=0  TranslationROffsetUnits=m  TranslationZOffset=0  TranslationZOffsetUnits=m  TranslationThetaOffset=0  TranslationThetaOffsetUnits=deg  RotationMethod=ArbitraryAxis  RotationAngleUnits=rad  RotationStandardAxis=+Z  RotationAngle=2.7352803968007873  RotationArbitraryAxis=[-0.20599796797350473 0.69194105138761164 0.69194105138761175]  FollAlignAxisA=+X  BaseAlignAxisA=+Y  FollAlignAxisB=+Y  BaseAlignAxisB=+Z  BlockFunction=simmechanics.library.frames_transforms.rigid_transform
  Transform4 : sm_lib/Frames and Transforms/Rigid Transform  TranslationMethod=Cartesian  TranslationLengthUnit=mm  TranslationStandardAxis=+Z  TranslationStandardOffset=0  TranslationCartesianOffset=[-16.089268306127362 -263.24103840837574 40.649351392904165]  TranslationROffset=0  TranslationROffsetUnits=m  TranslationZOffset=0  TranslationZOffsetUnits=m  TranslationThetaOffset=0  TranslationThetaOffsetUnits=deg  RotationMethod=ArbitraryAxis  RotationAngleUnits=rad  RotationStandardAxis=+Z  RotationAngle=3.1415926535897931  RotationArbitraryAxis=[-1.110223024625157e-16 0 1]  FollAlignAxisA=+X  BaseAlignAxisA=+Y  FollAlignAxisB=+Y  BaseAlignAxisB=+Z  BlockFunction=simmechanics.library.frames_transforms.rigid_transform
  Transform5 : sm_lib/Frames and Transforms/Rigid Transform  TranslationMethod=Cartesian  TranslationLengthUnit=mm  TranslationStandardAxis=+Z  TranslationStandardOffset=0  TranslationCartesianOffset=[-16.089268306127362 -199.74103840837569 40.649351392904165]  TranslationROffset=0  TranslationROffsetUnits=m  TranslationZOffset=0  TranslationZOffsetUnits=m  TranslationThetaOffset=0  TranslationThetaOffsetUnits=deg  RotationMethod=ArbitraryAxis  RotationAngleUnits=rad  RotationStandardAxis=+Z  RotationAngle=2.7352803968007873  RotationArbitraryAxis=[0.20599796797350473 0.69194105138761164 -0.69194105138761175]  FollAlignAxisA=+X  BaseAlignAxisA=+Y  FollAlignAxisB=+Y  BaseAlignAxisB=+Z  BlockFunction=simmechanics.library.frames_transforms.rigid_transform
  Transform6 : sm_lib/Frames and Transforms/Rigid Transform  TranslationMethod=Cartesian  TranslationLengthUnit=mm  TranslationStandardAxis=+Z  TranslationStandardOffset=0  TranslationCartesianOffset=[-16.089268306127391 11.758961591624317 40.649351392904165]  TranslationROffset=0  TranslationROffsetUnits=m  TranslationZOffset=0  TranslationZOffsetUnits=m  TranslationThetaOffset=0  TranslationThetaOffsetUnits=deg  RotationMethod=None  RotationAngleUnits=deg  RotationStandardAxis=+Z  RotationAngle=0  RotationArbitraryAxis=[0 0 1]  FollAlignAxisA=+X  BaseAlignAxisA=+Y  FollAlignAxisB=+Y  BaseAlignAxisB=+Z  BlockFunction=simmechanics.library.frames_transforms.rigid_transform
  uniball_Cuerpo_1_RIGID : Subsystem
  uniball_Cuerpo_2_RIGID : Subsystem
  F : PMIOPort  Port=1  Side=Left
  F1 : PMIOPort  Port=2  Side=Right
  connections:
  ReferenceFrame/RConn1 -- Transform/LConn1 -- Transform1/LConn1 -- Transform2/LConn1 -- Transform3/LConn1 -- Transform4/LConn1 -- Transform5/LConn1 -- Transform6/LConn1
  Transform/RConn1 -- F/RConn1
  Transform1/RConn1 -- F1/RConn1
  Acople_Antebrazo_RUniball_2_RIGID/LConn1 -- Transform2/RConn1
  Antebrazo_1_RIGID/LConn1 -- Transform3/RConn1
  Transform4/RConn1 -- uniball_Cuerpo_2_RIGID/LConn1
  Acople_Antebrazo_RUniball_1_RIGID/LConn1 -- Transform5/RConn1
  Transform6/RConn1 -- uniball_Cuerpo_1_RIGID/LConn1

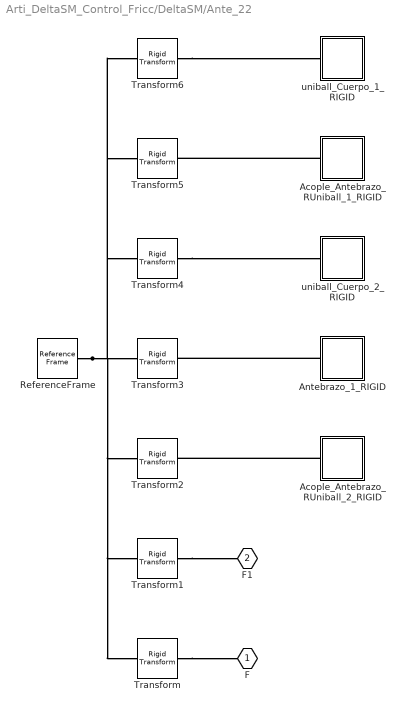
== system Arti_DeltaSM_Control_Fricc/DeltaSM/Ante_22 ==
  Acople_Antebrazo_RUniball_1_RIGID : Subsystem
  Acople_Antebrazo_RUniball_2_RIGID : Subsystem
  Antebrazo_1_RIGID : Subsystem
  ReferenceFrame : sm_lib/Frames and Transforms/Reference Frame  BlockFunction=simmechanics.library.frames_transforms.reference_frame
  Transform : sm_lib/Frames and Transforms/Rigid Transform  TranslationMethod=Cartesian  TranslationLengthUnit=mm  TranslationStandardAxis=+Z  TranslationStandardOffset=0  TranslationCartesianOffset=[-16.089268306127348 11.758961591624182 40.649351392904187]  TranslationROffset=0  TranslationROffsetUnits=m  TranslationZOffset=0  TranslationZOffsetUnits=m  TranslationThetaOffset=0  TranslationThetaOffsetUnits=deg  RotationMethod=ArbitraryAxis  RotationAngleUnits=rad  RotationStandardAxis=+Z  RotationAngle=0  RotationArbitraryAxis=[0 0 0]  FollAlignAxisA=+X  BaseAlignAxisA=+Y  FollAlignAxisB=+Y  BaseAlignAxisB=+Z  BlockFunction=simmechanics.library.frames_transforms.rigid_transform
  Transform1 : sm_lib/Frames and Transforms/Rigid Transform  TranslationMethod=Cartesian  TranslationLengthUnit=mm  TranslationStandardAxis=+Z  TranslationStandardOffset=0  TranslationCartesianOffset=[-16.089268306127391 -263.24103840837586 40.64935139290418]  TranslationROffset=0  TranslationROffsetUnits=m  TranslationZOffset=0  TranslationZOffsetUnits=m  TranslationThetaOffset=0  TranslationThetaOffsetUnits=deg  RotationMethod=ArbitraryAxis  RotationAngleUnits=rad  RotationStandardAxis=+Z  RotationAngle=0  RotationArbitraryAxis=[0 0 0]  FollAlignAxisA=+X  BaseAlignAxisA=+Y  FollAlignAxisB=+Y  BaseAlignAxisB=+Z  BlockFunction=simmechanics.library.frames_transforms.rigid_transform
  Transform2 : sm_lib/Frames and Transforms/Rigid Transform  TranslationMethod=Cartesian  TranslationLengthUnit=mm  TranslationStandardAxis=+Z  TranslationStandardOffset=0  TranslationCartesianOffset=[-16.089268306127391 -51.741038408375701 40.64935139290418]  TranslationROffset=0  TranslationROffsetUnits=m  TranslationZOffset=0  TranslationZOffsetUnits=m  TranslationThetaOffset=0  TranslationThetaOffsetUnits=deg  RotationMethod=ArbitraryAxis  RotationAngleUnits=rad  RotationStandardAxis=+Z  RotationAngle=2.7352803968007873  RotationArbitraryAxis=[-0.20599796797350467 0.69194105138761164 0.69194105138761164]  FollAlignAxisA=+X  BaseAlignAxisA=+Y  FollAlignAxisB=+Y  BaseAlignAxisB=+Z  BlockFunction=simmechanics.library.frames_transforms.rigid_transform
  Transform3 : sm_lib/Frames and Transforms/Rigid Transform  TranslationMethod=Cartesian  TranslationLengthUnit=mm  TranslationStandardAxis=+Z  TranslationStandardOffset=0  TranslationCartesianOffset=[-16.089268306127405 -227.74103840837577 40.64935139290418]  TranslationROffset=0  TranslationROffsetUnits=m  TranslationZOffset=0  TranslationZOffsetUnits=m  TranslationThetaOffset=0  TranslationThetaOffsetUnits=deg  RotationMethod=ArbitraryAxis  RotationAngleUnits=rad  RotationStandardAxis=+Z  RotationAngle=2.7352803968007873  RotationArbitraryAxis=[-0.20599796797350467 0.69194105138761164 0.69194105138761164]  FollAlignAxisA=+X  BaseAlignAxisA=+Y  FollAlignAxisB=+Y  BaseAlignAxisB=+Z  BlockFunction=simmechanics.library.frames_transforms.rigid_transform
  Transform4 : sm_lib/Frames and Transforms/Rigid Transform  TranslationMethod=Cartesian  TranslationLengthUnit=mm  TranslationStandardAxis=+Z  TranslationStandardOffset=0  TranslationCartesianOffset=[-16.089268306127391 -263.24103840837586 40.64935139290418]  TranslationROffset=0  TranslationROffsetUnits=m  TranslationZOffset=0  TranslationZOffsetUnits=m  TranslationThetaOffset=0  TranslationThetaOffsetUnits=deg  RotationMethod=ArbitraryAxis  RotationAngleUnits=rad  RotationStandardAxis=+Z  RotationAngle=3.1415926535897931  RotationArbitraryAxis=[-9.0856142054285235e-17 0 1]  FollAlignAxisA=+X  BaseAlignAxisA=+Y  FollAlignAxisB=+Y  BaseAlignAxisB=+Z  BlockFunction=simmechanics.library.frames_transforms.rigid_transform
  Transform5 : sm_lib/Frames and Transforms/Rigid Transform  TranslationMethod=Cartesian  TranslationLengthUnit=mm  TranslationStandardAxis=+Z  TranslationStandardOffset=0  TranslationCartesianOffset=[-16.089268306127405 -199.74103840837577 40.64935139290418]  TranslationROffset=0  TranslationROffsetUnits=m  TranslationZOffset=0  TranslationZOffsetUnits=m  TranslationThetaOffset=0  TranslationThetaOffsetUnits=deg  RotationMethod=ArbitraryAxis  RotationAngleUnits=rad  RotationStandardAxis=+Z  RotationAngle=2.7352803968007873  RotationArbitraryAxis=[0.20599796797350467 0.69194105138761164 -0.69194105138761164]  FollAlignAxisA=+X  BaseAlignAxisA=+Y  FollAlignAxisB=+Y  BaseAlignAxisB=+Z  BlockFunction=simmechanics.library.frames_transforms.rigid_transform
  Transform6 : sm_lib/Frames and Transforms/Rigid Transform  TranslationMethod=Cartesian  TranslationLengthUnit=mm  TranslationStandardAxis=+Z  TranslationStandardOffset=0  TranslationCartesianOffset=[-16.089268306127405 11.758961591624317 40.64935139290418]  TranslationROffset=0  TranslationROffsetUnits=m  TranslationZOffset=0  TranslationZOffsetUnits=m  TranslationThetaOffset=0  TranslationThetaOffsetUnits=deg  RotationMethod=None  RotationAngleUnits=deg  RotationStandardAxis=+Z  RotationAngle=0  RotationArbitraryAxis=[0 0 1]  FollAlignAxisA=+X  BaseAlignAxisA=+Y  FollAlignAxisB=+Y  BaseAlignAxisB=+Z  BlockFunction=simmechanics.library.frames_transforms.rigid_transform
  uniball_Cuerpo_1_RIGID : Subsystem
  uniball_Cuerpo_2_RIGID : Subsystem
  F : PMIOPort  Port=1  Side=Left
  F1 : PMIOPort  Port=2  Side=Right
  connections:
  ReferenceFrame/RConn1 -- Transform/LConn1 -- Transform1/LConn1 -- Transform2/LConn1 -- Transform3/LConn1 -- Transform4/LConn1 -- Transform5/LConn1 -- Transform6/LConn1
  Transform/RConn1 -- F/RConn1
  Transform1/RConn1 -- F1/RConn1
  Acople_Antebrazo_RUniball_2_RIGID/LConn1 -- Transform2/RConn1
  Antebrazo_1_RIGID/LConn1 -- Transform3/RConn1
  Transform4/RConn1 -- uniball_Cuerpo_2_RIGID/LConn1
  Acople_Antebrazo_RUniball_1_RIGID/LConn1 -- Transform5/RConn1
  Transform6/RConn1 -- uniball_Cuerpo_1_RIGID/LConn1

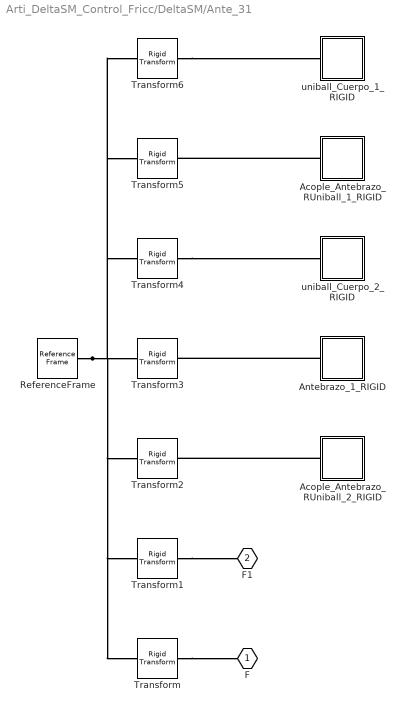
== system Arti_DeltaSM_Control_Fricc/DeltaSM/Ante_31 ==
  Acople_Antebrazo_RUniball_1_RIGID : Subsystem
  Acople_Antebrazo_RUniball_2_RIGID : Subsystem
  Antebrazo_1_RIGID : Subsystem
  ReferenceFrame : sm_lib/Frames and Transforms/Reference Frame  BlockFunction=simmechanics.library.frames_transforms.reference_frame
  Transform : sm_lib/Frames and Transforms/Rigid Transform  TranslationMethod=Cartesian  TranslationLengthUnit=mm  TranslationStandardAxis=+Z  TranslationStandardOffset=0  TranslationCartesianOffset=[-16.089268306127362 11.758961591624349 40.649351392904215]  TranslationROffset=0  TranslationROffsetUnits=m  TranslationZOffset=0  TranslationZOffsetUnits=m  TranslationThetaOffset=0  TranslationThetaOffsetUnits=deg  RotationMethod=ArbitraryAxis  RotationAngleUnits=rad  RotationStandardAxis=+Z  RotationAngle=0  RotationArbitraryAxis=[0 0 0]  FollAlignAxisA=+X  BaseAlignAxisA=+Y  FollAlignAxisB=+Y  BaseAlignAxisB=+Z  BlockFunction=simmechanics.library.frames_transforms.rigid_transform
  Transform1 : sm_lib/Frames and Transforms/Rigid Transform  TranslationMethod=Cartesian  TranslationLengthUnit=mm  TranslationStandardAxis=+Z  TranslationStandardOffset=0  TranslationCartesianOffset=[-16.089268306127391 -263.24103840837569 40.649351392904222]  TranslationROffset=0  TranslationROffsetUnits=m  TranslationZOffset=0  TranslationZOffsetUnits=m  TranslationThetaOffset=0  TranslationThetaOffsetUnits=deg  RotationMethod=ArbitraryAxis  RotationAngleUnits=rad  RotationStandardAxis=+Z  RotationAngle=0  RotationArbitraryAxis=[0 0 0]  FollAlignAxisA=+X  BaseAlignAxisA=+Y  FollAlignAxisB=+Y  BaseAlignAxisB=+Z  BlockFunction=simmechanics.library.frames_transforms.rigid_transform
  Transform2 : sm_lib/Frames and Transforms/Rigid Transform  TranslationMethod=Cartesian  TranslationLengthUnit=mm  TranslationStandardAxis=+Z  TranslationStandardOffset=0  TranslationCartesianOffset=[-16.089268306127376 -51.741038408375701 40.649351392904194]  TranslationROffset=0  TranslationROffsetUnits=m  TranslationZOffset=0  TranslationZOffsetUnits=m  TranslationThetaOffset=0  TranslationThetaOffsetUnits=deg  RotationMethod=ArbitraryAxis  RotationAngleUnits=rad  RotationStandardAxis=+Z  RotationAngle=2.7352803968007873  RotationArbitraryAxis=[-0.20599796797350475 0.69194105138761153 0.69194105138761164]  FollAlignAxisA=+X  BaseAlignAxisA=+Y  FollAlignAxisB=+Y  BaseAlignAxisB=+Z  BlockFunction=simmechanics.library.frames_transforms.rigid_transform
  Transform3 : sm_lib/Frames and Transforms/Rigid Transform  TranslationMethod=Cartesian  TranslationLengthUnit=mm  TranslationStandardAxis=+Z  TranslationStandardOffset=0  TranslationCartesianOffset=[-16.089268306127405 -227.74103840837572 40.649351392904194]  TranslationROffset=0  TranslationROffsetUnits=m  TranslationZOffset=0  TranslationZOffsetUnits=m  TranslationThetaOffset=0  TranslationThetaOffsetUnits=deg  RotationMethod=ArbitraryAxis  RotationAngleUnits=rad  RotationStandardAxis=+Z  RotationAngle=2.7352803968007873  RotationArbitraryAxis=[-0.20599796797350475 0.69194105138761153 0.69194105138761164]  FollAlignAxisA=+X  BaseAlignAxisA=+Y  FollAlignAxisB=+Y  BaseAlignAxisB=+Z  BlockFunction=simmechanics.library.frames_transforms.rigid_transform
  Transform4 : sm_lib/Frames and Transforms/Rigid Transform  TranslationMethod=Cartesian  TranslationLengthUnit=mm  TranslationStandardAxis=+Z  TranslationStandardOffset=0  TranslationCartesianOffset=[-16.089268306127391 -263.24103840837569 40.649351392904222]  TranslationROffset=0  TranslationROffsetUnits=m  TranslationZOffset=0  TranslationZOffsetUnits=m  TranslationThetaOffset=0  TranslationThetaOffsetUnits=deg  RotationMethod=ArbitraryAxis  RotationAngleUnits=rad  RotationStandardAxis=+Z  RotationAngle=3.1415926535897931  RotationArbitraryAxis=[-1.1102230246251565e-16 0 1]  FollAlignAxisA=+X  BaseAlignAxisA=+Y  FollAlignAxisB=+Y  BaseAlignAxisB=+Z  BlockFunction=simmechanics.library.frames_transforms.rigid_transform
  Transform5 : sm_lib/Frames and Transforms/Rigid Transform  TranslationMethod=Cartesian  TranslationLengthUnit=mm  TranslationStandardAxis=+Z  TranslationStandardOffset=0  TranslationCartesianOffset=[-16.089268306127376 -199.74103840837572 40.649351392904208]  TranslationROffset=0  TranslationROffsetUnits=m  TranslationZOffset=0  TranslationZOffsetUnits=m  TranslationThetaOffset=0  TranslationThetaOffsetUnits=deg  RotationMethod=ArbitraryAxis  RotationAngleUnits=rad  RotationStandardAxis=+Z  RotationAngle=2.7352803968007873  RotationArbitraryAxis=[0.20599796797350475 0.69194105138761153 -0.69194105138761164]  FollAlignAxisA=+X  BaseAlignAxisA=+Y  FollAlignAxisB=+Y  BaseAlignAxisB=+Z  BlockFunction=simmechanics.library.frames_transforms.rigid_transform
  Transform6 : sm_lib/Frames and Transforms/Rigid Transform  TranslationMethod=Cartesian  TranslationLengthUnit=mm  TranslationStandardAxis=+Z  TranslationStandardOffset=0  TranslationCartesianOffset=[-16.089268306127405 11.758961591624331 40.649351392904208]  TranslationROffset=0  TranslationROffsetUnits=m  TranslationZOffset=0  TranslationZOffsetUnits=m  TranslationThetaOffset=0  TranslationThetaOffsetUnits=deg  RotationMethod=None  RotationAngleUnits=deg  RotationStandardAxis=+Z  RotationAngle=0  RotationArbitraryAxis=[0 0 1]  FollAlignAxisA=+X  BaseAlignAxisA=+Y  FollAlignAxisB=+Y  BaseAlignAxisB=+Z  BlockFunction=simmechanics.library.frames_transforms.rigid_transform
  uniball_Cuerpo_1_RIGID : Subsystem
  uniball_Cuerpo_2_RIGID : Subsystem
  F : PMIOPort  Port=1  Side=Left
  F1 : PMIOPort  Port=2  Side=Right
  connections:
  ReferenceFrame/RConn1 -- Transform/LConn1 -- Transform1/LConn1 -- Transform2/LConn1 -- Transform3/LConn1 -- Transform4/LConn1 -- Transform5/LConn1 -- Transform6/LConn1
  Transform/RConn1 -- F/RConn1
  Transform1/RConn1 -- F1/RConn1
  Acople_Antebrazo_RUniball_2_RIGID/LConn1 -- Transform2/RConn1
  Antebrazo_1_RIGID/LConn1 -- Transform3/RConn1
  Transform4/RConn1 -- uniball_Cuerpo_2_RIGID/LConn1
  Acople_Antebrazo_RUniball_1_RIGID/LConn1 -- Transform5/RConn1
  Transform6/RConn1 -- uniball_Cuerpo_1_RIGID/LConn1
